simulink model "DRemoveConRR"  (Simulink 7.8)
settings: Solver=ode45  StartTime=0.0  StopTime=10.0  RelTol=1e-3
settings Model: Creator=Arne Haber  LastModifiedBy=fkolass

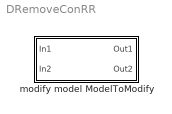
== system DRemoveConRR ==
  modify model ModelToModify : Subsystem

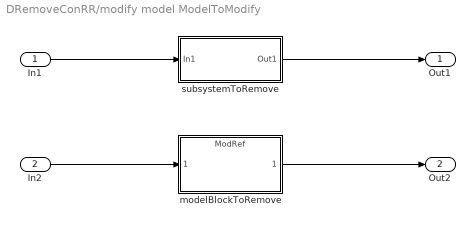
== system DRemoveConRR/modify model ModelToModify ==
  In1 : Inport
  In2 : Inport  Port=2
  modelBlockToRemove : ModelReference  ModelNameDialog=ModRef  SimulationMode=Normal  ModelReferenceVersion=1.1  CopyOfModelName=ModRef  DefaultDataLogging=on
  subsystemToRemove : Subsystem
  Out1 : Outport
  Out2 : Outport  Port=2
  wires:
  In1/1 -> subsystemToRemove/1(In1)
  In2/1 -> modelBlockToRemove/1
  subsystemToRemove/1(Out1) -> Out1/1
  modelBlockToRemove/1 -> Out2/1

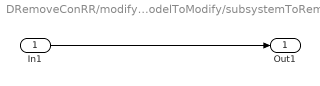
== system DRemoveConRR/modify model ModelToModify/subsystemToRemove ==
  In1 : Inport
  Out1 : Outport
  wires:
  In1/1 -> Out1/1
